simulink library "biogas"  (Simulink 7.8)
settings: Solver=ode45  StartTime=0.0  StopTime=10.0  RelTol=1e-3
undefined symbols (not defined in the file or in its folder): adm1_loadfcn, appendDATA, biogas, Callback_ADM1_gui, configdivider, configmixer, datasourcetypes, DEBUG, deltatime, gas2bhkwsplittypes, hydraulic_delay_loadfcn, init_biogas_plant_mdl, initstatetypes, kalman_loadfcn, lda_state_estimator_loadfcn, plant, plant_network, pump_energy_loadfcn, pump_stream_loadfcn, sensors, substrate, substrate_mixer_digester_loadfcn, substrate_network, volumeflowtypes
libraries: biogas x8, simulink x5
(part 1 of 2)
Description:
  | This library consists of blocks, which are useful for biogas plant modeling.
  | It belongs to the 'Biogas Plant Modeling' toolbox.
  | 
  | The library consists of seven sublibraries.
  | The most important blocks in these sublibraries are:
  | 
  | - Anaerobic Digestion Models
  | - Biogas Plant Components
  | - Commonly used blocks
  | - Optimization
  | - Sensors
  | - Simba Biogas Blocks
  | - Substrate Sources
settings Model: Creator=Daniel Gaida  LastModifiedBy=Daniel

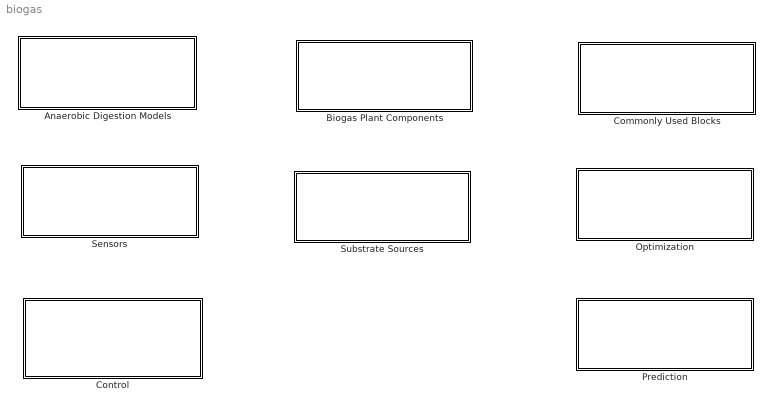
== system biogas ==
  Anaerobic Digestion Models : Subsystem  Description=This sub library contains blocks which model the anaerobic digestion process of a digester on a biogas plant. It includes the famous Anaerobic Digestion Model No.1 (ADM1).
      mask Type: Anaerobic Digestion Models
      mask Display: disp('Anaerobic Digestion Models')
  Biogas Plant Components : Subsystem  Description=This sub library contains blocks of components which are usually found on a biogas plant. Among these components are pump, heating, chp, mixer, etc...
      mask Type: Biogas Plant Components
      mask Display: disp('Biogas Plant Components')
  Commonly Used Blocks : Subsystem  Description=This sub library contains blocks, which are used very often modeling biogas plants.
      mask Type: Commonly Used Blocks
      mask Display: disp('Commonly Used Blocks')
  Control : Subsystem
      mask Display: disp('Control')
  Optimization : Subsystem
      mask Display: disp('Optimization')
  Prediction : Subsystem
      mask Display: disp('Prediction')
  Sensors : Subsystem  Description=This sub library contains measurement sensors, often installed on biogas plants.  mask(Sensors){d=0}
      mask help:
      | There is no public access to the Sensors using the Simulink Library Browser.
      | All sensors are integrated in other blocks, such as the ADM and substrate mixer blocks.
      mask Display: disp('Sensors')
  Substrate Sources : Subsystem
      mask Display: disp('Substrate Sources')

== system biogas/Anaerobic Digestion Models ==
  note: Callback_ADM1_gui('InitFcn', 'ADM1DE');
      | Callback_ADM1_gui('LoadFcn', 'ADM1DE');
      | Callback_ADM1_gui('ModelCloseFcn', 'ADM1DE');
      | Callback_ADM1_gui('StopFcn', 'ADM1DE');
  ADM1DE Linearized with GUI : Subsystem  LoadFcn=Callback_ADM1_gui('LoadFcn', 'ADM1DE', plant, DEBUG);  InitFcn=Callback_ADM1_gui('InitFcn', 'ADM1DE', plant, DEBUG);  StopFcn=Callback_ADM1_gui('StopFcn', 'ADM1DE', plant, DEBUG);  mask(ADM1 implementation with GUI (clone of Simba's ADM1xp model)){fermenter_name=--- Bitte Fermenter wählen ---, initstate_type=user, datasource_type=file, savestate=off, isload=off, isbeingloaded=off, isbeingclosed=off, DEBUG_DISP=off}
      mask prompts: fermenter_name "name of the fermenter (fermenter_name)"; initstate_type "initial state type (initstate_type)"; datasource_type "source for the initial state (datasource_type)"; savestate "save final state in variable/file (overwrite existing type, except default, than save in user)"; isload "if checked then this block is loaded"; isbeingloaded "if checked then this block is actually being loaded"; isbeingclosed "if checked then this block is actually being closed"; DEBUG_DISP "if checked then DEBUG_DISP modus is on for this block"
      mask help:
      | This block contains the block 'ADM1DE' and some measurement sensors like the pH, TS, SS, biogas and volumeflow sensor. These measurements are presented on a GUI, which is, in DEBUG mode, shown during the simulation.
      |
      | This block is implemented as the clone of the 'ADM1xp with GUI' block and can be used as an alternative, when Simba can't be used. For steady state simulations the gained results should be exactly the same.
      mask init:
      | if (DEBUG_DISP)
      |     disp(['Initialization commands of block ', gcb]);
      | end
      | 
      | values= get_param(gcb, 'MaskValues');
      | 
      | if isempty(values)
      |     error('Could not read the parameter MaskValues of block %s!', gcb);
      | end
      |     
      | if strcmp( char(values(5,1)), 'off' )
      | 
      |     if strcmp( char(values(6,1)), 'off' )
      |         
      |         if strcmp( char(values(7,1)), 'off' )
      |             
      |             Callback_ADM1_gui('LoadFcn', 'ADM1DE', plant, DEBUG, DEBUG_DISP);
      |             
      |         end
      |         
      |     end
      | 
      | else
      | 
      |     if strcmp( char(values(7,1)), 'off' )
      |             
      |         adm1_with_gui_setmasks(1,2,3,4);
      |         
      |     end
      | 
      | end
      | 
      | clear values;
      settings: ModelCloseFcn=Callback_ADM1_gui('ModelCloseFcn', 'ADM1DE', plant, DEBUG);
      mask StyleString: popup(--- Bitte Fermenter wählen ---),popup(--- Bitte Startzustandstyp wählen ---|default|random|user),popup(--- Bitte Datenquelle wählen ---|file|workspace|extern|modelworkspace),checkbox,checkbox,checkbox,checkbox,checkbox
      mask CallbackString:
      | values= get_param(gcb, 'MaskValues');
      | 
      | if isempty(values)
      |     error('Could not read the parameter MaskValues of block %s!', gcb);
      | end
      | 
      | if strcmp( char(values(5,1)), 'on' )
      | 
      |     display_selected_fermenter(1, 0.7);
      | 
      | end
      | 
      | clear values;
      | |
      | createinitstatetypepopup(2, 0);
      | |
      | createdatasourcetypepopup(3, 0);
      | |||||
      mask Display:
      | image(imread('icon_s6_digester','bmp'),'center')
      | port_label('input', 1, 'Qin', ...
      |     'texmode', 'on')
      | port_label('output', 1, 'Gas [m^3/d]')
      | port_label('output', 2, 'Qe')
      | port_label('output', 3, 'int.vars')
      | text(0.5, 7.0e-001, '--- Bitte Fermenter wählen ---', 'horizontalAlignment', 'center')
  ADM1DE with GUI : Subsystem  LoadFcn=Callback_ADM1_gui('LoadFcn', 'ADM1DE', plant, DEBUG);  InitFcn=Callback_ADM1_gui('InitFcn', 'ADM1DE', plant, DEBUG);  StopFcn=Callback_ADM1_gui('StopFcn', 'ADM1DE', plant, DEBUG);  mask(ADM1 implementation with GUI (clone of Simba's ADM1xp model)){fermenter_name=--- Bitte Fermenter wählen ---, initstate_type=user, datasource_type=file, savestate=off, isload=off, isbeingloaded=off, isbeingclosed=off, DEBUG_DISP=off, heating_onoff=off}
      mask prompts: fermenter_name "name of the fermenter (fermenter_name)"; initstate_type "initial state type (initstate_type)"; datasource_type "source for the initial state (datasource_type)"; savestate "save final state in variable/file (overwrite existing type, except default, than save in user)"; isload "if checked then this block is loaded"; isbeingloaded "if checked then this block is actually being loaded"; isbeingclosed "if checked then this block is actually being closed"; DEBUG_DISP "if checked then DEBUG_DISP modus is on for this block"; heating_onoff "check if heating is switched on, uncheck if digester is not heated"
      mask help:
      | This block contains the block 'ADM1DE' and some measurement sensors like the pH, TS, SS, biogas and volumeflow sensor. These measurements are presented on a GUI, which is, in DEBUG mode, shown during the simulation.
      |
      | This block is implemented as the clone of the 'ADM1xp with GUI' block and can be used as an alternative, when Simba can't be used. For steady state simulations the gained results should be exactly the same.
      mask init: same as biogas/Anaerobic Digestion Models/ADM1DE Linearized with GUI
      settings: ModelCloseFcn=Callback_ADM1_gui('ModelCloseFcn', 'ADM1DE', plant, DEBUG);
      mask StyleString: popup(--- Bitte Fermenter wählen ---),popup(--- Bitte Startzustandstyp wählen ---|default|random|user),popup(--- Bitte Datenquelle wählen ---|file|workspace|extern|modelworkspace),checkbox,checkbox,checkbox,checkbox,checkbox,checkbox
      mask CallbackString:
      | values= get_param(gcb, 'MaskValues');
      | 
      | if isempty(values)
      |     error('Could not read the parameter MaskValues of block %s!', gcb);
      | end
      | 
      | if strcmp( char(values(5,1)), 'on' )
      | 
      |     display_selected_fermenter(1, 0.7);
      | 
      | end
      | 
      | clear values;
      | |
      | createinitstatetypepopup(2, 0);
      | |
      | createdatasourcetypepopup(3, 0);
      | ||||||
      mask Display:
      | image(imread('icon_s6_digester','bmp'),'center')
      | port_label('input', 1, 'Qin', ...
      |     'texmode', 'on')
      | port_label('output', 1, 'Gas [m^3/d]')
      | port_label('output', 2, 'Qe')
      | text(0.5, 7.0e-001, '--- Bitte Fermenter wählen ---', 'horizontalAlignment', 'center')
  Internal : Subsystem
      mask Type: Internal Blocks
      mask Description: There is no public access to this group of blocks.
      mask Display: disp('No Public Access')

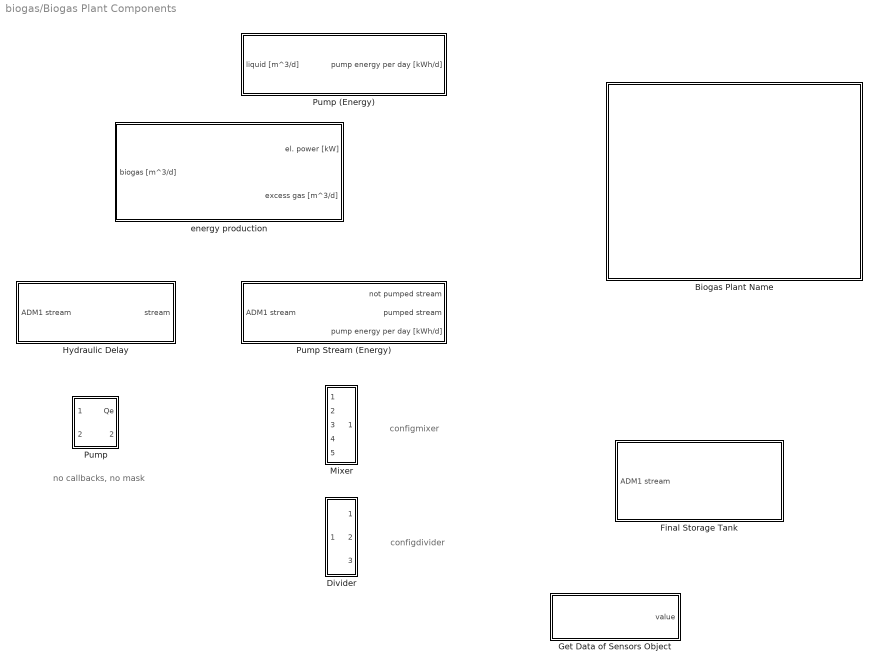
== system biogas/Biogas Plant Components ==
  note: no callbacks, no mask
  note: configmixer
  note: configdivider
  Biogas Plant Name : Subsystem  LoadFcn=init_biogas_plant_mdl();  InitFcn=init_biogas_plant_mdl();  mask(Biogas Plant    ){plant_name=plantname, debug=off, timegrid=min, timevalue=1}
      mask prompts: plant_name "Enter the name of the biogas plant (has to be identical with plant.name) (e.g. sunderhook):"; debug "Run model in DEBUG mode"; timegrid "In DEBUG mode much data is saved to file and workspace. Define here the unit of the timegrid"; timevalue "Select the number multiplied by the unit"
      mask help: This block serves as a framework for modeling your biogas plant. If you build a new biogas plant this block should be the first block you have to insert in the simulink model. Under the mask of this block you can then model your biogas plant by inserting digesters, chp's, substrate sources, pumps, etc...
      mask init:
      | values= get_param(gcb, 'MaskValues');
      | 
      | if ~isempty(values)
      | 
      |     img_filename= sprintf('plant_%s.jpg', char(values(1,1)));
      | 
      |     if ~exist(img_filename, 'file')
      |         warning(['Could not find the image ''', img_filename, ...
      |                 '''! Using the image ''plant_plantname.jpg'' instead!']);
      |         img_filename= 'plant_plantname.jpg';
      |     end
      |     
      | end
      mask StyleString: edit,checkbox,popup(day|hour|min|sec|each),popup(1)
      mask CallbackString:
      | init_biogas_plant_mdl();
      | |createtimevaluepopup();|createtimevaluepopup();|createtimevaluepopup();
      mask Display: image(imread(img_filename));
  Divider : Subsystem  InitFcn=configdivider();  mask(ADM1 Stream Divider){n_outputs=3, splitVector=[0.25, 0.5, 0.25, 0.1]}
      mask prompts: n_outputs "Number of Outflows"; splitVector "How should the stream be divided? Give a vector: e.g. [0.25, 0.5, 0.25], if number of Outputs = 3"
      mask help: This block divides the ADM1 stream.
      mask init:
      | %n_outputs=max(2,n_outputs);
      | if n_outputs == 1
      |     yi= 0.5;
      |     
      |     lb_x= 0;
      |     lb_y= -0.5;
      |     ub_x= 0.5;
      |     ub_y= 1.5;
      | else
      |     yi=[0:n_outputs-1]/(n_outputs-1);
      |     
      |     lb_x= 0;
      |     lb_y= -0.5/(n_outputs-1);
      |     ub_x= 0.5;
      |     ub_y= 1 + 0.5/(n_outputs-1);
      | end
      | 
      | x=[];y=[];
      | 
      | for i=1:n_outputs,
      |    
      |     x=[x; 0.0;0.3; 0.5;0.3; 0.0];
      |     y=[y;0.5; yi(i);yi(i);yi(i);0.5];
      |   
      | end;
      | 
      | configdivider();
      mask Help: eval('web( ''html/divider.html'', ''-helpbrowser'')')
      mask Display: plot(lb_x, lb_y, ub_x, ub_y, x, y);
  Final Storage Tank : Subsystem
      mask Type: Final Storage Tank
      mask Description: This block models the final storage tank.
      mask Display:
      | image(imread('images/final_storage_tank.bmp'))
      | color('red')
      | 
      | port_label('input', 1, 'ADM1 stream')
  Get Data of Sensors Object : Subsystem  mask(Get Data of Sensors Object){processvalue='Q_main_2', id_in_array='', index=0, noisy=off}
      mask prompts: processvalue "process value id"; index "index in sensor (0, 1, 2, ...)"; noisy "noisy sensor values"
      mask help: This block returns the current value of the specified process value.
      settings: AttributesFormatString=%<processvalue>
  Hydraulic Delay : Subsystem  LoadFcn=hydraulic_delay_loadfcn();  mask(Hydraulic Delay){fermenter_name_start=--- Bitte Fermenter wählen ---, fermenter_name_destiny=--- Bitte Fermenter wählen ---, initstate_type=--- Bitte Startzustandstyp wählen ---, datasource_type=--- Bitte Datenquelle wählen ---, savestate=off, time_constant=10, V_min=100, isload=on, isbeingloaded=off, isbeingclosed=off, DEBUG_DISP=off}
      mask prompts: fermenter_name_start "name of the start fermenter (fermenter_name_start)"; fermenter_name_destiny "name of the destiny fermenter (fermenter_name_destiny)"; initstate_type "initial state type (initstate_type)"; datasource_type "source for the initial state (datasource_type)"; savestate "save final state in variable/file (overwrite existing type, except default, than save in user)"; time_constant "Time constant [d]"; V_min "Minimum Volume [m^3]"; isload "if checked then this block is loaded"; isbeingloaded "if checked then this block is actually being loaded"; isbeingclosed "if checked then this block is actually being closed"; DEBUG_DISP "if checked then DEBUG_DISP modus is on for this block"
      mask help:
      | This block implements a hydraulic delay (first order storage).
      |
      | It is mainly used to avoid numerical loops. Most of the time they appear when substrate is pumped in a loop. Out of this reason the block 'Pump Stream (Energy)' consists this hydraulic delay block, such that, if you want to pump substrate in a loop, you don't have to bother about numerical loops. To summarize, normally you don't have to use this block.
      mask init:
      | x=[0:5:50];
      | y=ones(1,size(x,1))-exp(-x/5);
      | y=y*70;
      | 
      | 
      | if ~isempty(bdroot)
      |     hws= get_param(bdroot, 'modelworkspace');
      | else
      |     hws= [];
      | end
      | 
      | if ~isempty(hws)
      |    
      | if DEBUG_DISP       
      |     disp(['Initialization commands of block ', gcb]);
      | end
      | 
      | values= get_param(gcb, 'MaskValues');
      | 
      | if isempty(values)
      |     error('Could not read the parameter MaskValues of block %s!', gcb);
      | end
      |     
      | if strcmp( char(values(8,1)), 'off' )
      | 
      |     if strcmp( char(values(9,1)), 'off' )
      |         
      |         if strcmp( char(values(10,1)), 'off' )
      |          
      |             hydraulic_delay_loadfcn(DEBUG_DISP);
      |             
      |         end
      |         
      |     end
      | 
      | end
      | 
      | end
      | 
      | clear values hws;
      settings: ModelCloseFcn=hydraulic_delay_closefcn();
      mask Help: eval('web( ''html/hydraulic_delay.html'', ''-helpbrowser'')')
      mask StyleString: popup(--- Bitte Fermenter wählen ---),popup(--- Bitte Fermenter wählen ---),popup(--- Bitte Startzustandstyp wählen ---|default|random|user),popup(--- Bitte Datenquelle wählen ---|file|workspace|extern|modelworkspace),checkbox,edit,edit,checkbox,checkbox,checkbox,checkbox
      mask CallbackString:
      | values= get_param(gcb, 'MaskValues');
      | 
      | if isempty(values)
      |     error('Could not read the parameter MaskValues of block %s!', gcb);
      | end
      | 
      | if strcmp( char(values(8,1)), 'on' )
      | 
      |     display_selected_fermenter(1, 0.8);
      | 
      | end
      | 
      | clear values;
      | |
      | values= get_param(gcb, 'MaskValues');
      | 
      | if isempty(values)
      |     error('Could not read the parameter MaskValues of block %s!', gcb);
      | end
      | 
      | if strcmp( char(values(8,1)), 'on' )
      | 
      |     display_selected_fermenter(2, 0.4);
      | 
      | end
      | 
      | clear values;
      | |
      | values= get_param(gcb, 'MaskValues');
      | 
      | if isempty(values)
      |     error('Could not read the parameter MaskValues of block %s!', gcb);
      | end
      | 
      | if strcmp( char(values(8,1)), 'on' )
      | 
      |     createvolumeflowtypepopup(3, 0);
      | 
      | end
      | 
      | clear values;
      | |
      | values= get_param(gcb, 'MaskValues');
      | 
      | if isempty(values)
      |     error('Could not read the parameter MaskValues of block %s!', gcb);
      | end
      | 
      | if strcmp( char(values(8,1)), 'on' )
      | 
      |     createdatasourcetypepopup(4, 0);
      | 
      | end
      | 
      | clear values;
      | |||||||
      mask Display:
      | plot(0,0,100,100,[15,15,85],[85,15,15],...
      |      x+15,y+15,[0,10],[15,0]);
      |  text(0.5, 8.0e-001, '--- Bitte Fermenter wählen ---', 'horizontalAlignment', 'center')
      |  text(0.5, 4.0e-001, '--- Bitte Fermenter wählen ---', 'horizontalAlignment', 'center')
  Mixer : Subsystem  InitFcn=configmixer();  mask(Substrate Mixer){n_inputs=5}
      mask prompts: n_inputs "Number of Inflows"
      mask help: This block mixes the substrate flow.
      mask init:
      | %n_inputs=max(2,n_inputs);
      | 
      | if n_inputs == 1
      |     yi= 0.5;
      |     
      |     lb_x= 0;
      |     lb_y= -0.5;
      |     ub_x= 0.5;
      |     ub_y= 1.5;
      | else
      |     yi=[0:n_inputs-1]/(n_inputs-1);
      |     
      |     lb_x= 0;
      |     lb_y= -0.5/(n_inputs-1);
      |     ub_x= 0.5;
      |     ub_y= 1+0.5/(n_inputs-1);
      | end
      | 
      | x=[];y=[];
      | for i=1:n_inputs,
      |    
      |     x=[x; 0.5;0.2; 0.0;0.2; 0.5];
      |     y=[y;0.5; yi(i);yi(i);yi(i);0.5];
      |   
      | end;
      | 
      | configmixer();
      mask Help: eval('web( ''html/mixer.html'', ''-helpbrowser'')')
      mask Display: plot(lb_x, lb_y, ub_x, ub_y, x, y);
  Pump : Subsystem  mask(Pump){}
      mask help:
      | Pump a separated substrate stream flow.
      |
      | Remark: For the most purposes the 'Pump Stream (Energy)' block should be a better alternative.
      mask init:
      | x1=[10,90];
      | y1=[75,75];
      | x2=[30,40];
      | y2=[75,65];
      | x3=[65,80,90];
      | y3=[40,25,25];
      | 
      | ori=get_param(gcb,'orientation');
      | 
      | if strcmp(ori,'left')
      |     x1=100-x1;
      |     x2=100-x2;
      |     x3=100-x3;
      | elseif strcmp(ori,'down')
      |     xt=x1;
      |     x1=100-y1;
      |     y1=100-xt;
      |     xt=x2;
      |     x2=100-y2;
      |     y2=100-xt;
      |     xt=x3;
      |     x3=100-y3;
      |     y3=100-xt;
      | elseif strcmp(ori,'up')
      |     xt=x1;
      |     x1=100-y1;
      |     y1=xt;
      |     xt=x2;
      |     x2=100-y2;
      |     y2=xt;
      |     xt=x3;
      |     x3=100-y3;
      |     y3=xt;
      | end
      mask Display: plot(0,0,100,100,x1,y1,x2,y2,x3,y3,[0,20],[20,0]);disp('P')
  Pump (Energy) : Subsystem  LoadFcn=pump_energy_loadfcn();  mask(Pump (Energy)){fermenter_name=--- Bitte Fermenter wählen ---, h_friction=1.0, isload=off, isbeingloaded=off, isbeingclosed=off, DEBUG_DISP=off}
      mask prompts: fermenter_name "name of the fermenter (fermenter_name)"; isload "if checked then this block is loaded"; isbeingloaded "if checked then this block is actually being loaded"; isbeingclosed "if checked then this block is actually being closed"; DEBUG_DISP "if checked then DEBUG_DISP modus is on for this block"
      mask help:
      | This block calculates the power used to pump the substrate mix, whose volumeflow is given on the input.
      |
      | Remark: If you want to pump a stream, then use the block 'Pump' or even better the block 'Pump Stream (Energy)'.
      mask init:
      | if DEBUG_DISP
      |     disp(['Initialization commands of block ', gcb]);
      | end
      | 
      | values= get_param(gcb, 'MaskValues');
      | 
      | if isempty(values)
      |     error('Could not read the parameter MaskValues of block %s!', gcb);
      | end
      |     
      | if strcmp( char(values(3,1)), 'off' )
      | 
      |     if strcmp( char(values(4,1)), 'off' )
      |         
      |         if strcmp( char(values(5,1)), 'off' )
      |          
      |             pump_energy_loadfcn(DEBUG_DISP);
      |             
      |         end
      |         
      |     end
      | 
      | end
      | 
      | clear values;
      settings: ModelCloseFcn=pump_energy_closefcn();
      mask Help: eval('web( ''html/pump.html'', ''-helpbrowser'')')
      mask StyleString: popup(--- Bitte Fermenter wählen ---),edit,checkbox,checkbox,checkbox,checkbox
      mask CallbackString:
      | values= get_param(gcb, 'MaskValues');
      | 
      | if isempty(values)
      |     error('Could not read the parameter MaskValues of block %s!', gcb);
      | end
      | 
      | if strcmp( char(values(3,1)), 'on' )
      | 
      |     display_selected_fermenter(1, 0.3);
      | 
      | end
      | 
      | clear values;
      | 
      | |||||
      mask Display:
      | image(imread('images/Pumpe.jpg'))
      | color('red')
      | 
      | port_label('input', 1, 'liquid [m^3/d]', ...
      |     'texmode', 'on')
      | port_label('output', 1, 'pump energy per day [kWh/d]')
  Pump Stream (Energy) : Subsystem  LoadFcn=pump_stream_loadfcn();  mask(Pump Stream (Energy)){fermenter_name_start=--- Bitte Fermenter wählen ---, fermenter_name_destiny=--- Bitte Fermenter wählen ---, volumeflow_type=const, datasource_type=workspace, h_friction=1.0, hyd_delay=on, initstate_type=default, savestate=on, time_constant=1/24/30, V_min=100, isload=off, isbeingloaded=off, isbeingclosed=off, DEBUG_DISP=off}
      mask prompts: fermenter_name_start "name of the start fermenter (fermenter_name_start)"; fermenter_name_destiny "name of the destiny fermenter (fermenter_name_destiny)"; volumeflow_type "volumeflow_type : type of the volume flow pump data"; datasource_type "source for the volumeflow (datasource_type)"; hyd_delay "avoid algebraic loop by inserting an hydraulic delay"; initstate_type "initial state type (initstate_type)"; savestate "save final state in variable/file (overwrite existing type, except default, then save in user)"; time_constant "Time constant [d]"; V_min "Minimum Volume [m^3]"; isload "if checked then this block is loaded"; isbeingloaded "if checked then this block is actually being loaded"; isbeingclosed "if checked then this block is actually being closed"; DEBUG_DISP "if checked then DEBUG_DISP modus is on for this block"
      mask help: This block pumps a substrate stream and calculates the power used to pump the substrate stream. To avoid numerical loops this block contains the 'Hydraulic Delay' block, which can be inserted or deleted via the gui of this block.
      mask init:
      | pump_stream_init_comm(DEBUG_DISP);
      settings: ModelCloseFcn=pump_stream_closefcn();
      mask Help: eval('web( ''html/pump_stream.html'', ''-helpbrowser'')')
      mask StyleString: popup(--- Bitte Fermenter wählen ---),popup(--- Bitte Fermenter wählen ---),popup(--- Bitte Zulauftyp wählen ---|const|random|user),popup(--- Bitte Datenquelle wählen ---|file|workspace|extern|modelworkspace),edit,checkbox,popup(--- Bitte Startzustandstyp wählen ---|default|random|user),checkbox,edit,edit,checkbox,checkbox,checkbox,checkbox
      mask CallbackString:
      | values= get_param(gcb, 'MaskValues');
      | 
      | if isempty(values)
      |     error('Could not read the parameter MaskValues of block %s!', gcb);
      | end
      | 
      | if strcmp( char(values(11,1)), 'on' )
      | 
      |     display_selected_fermenter(1, 0.8);
      | 
      | end
      | 
      | clear values;
      | |
      | values= get_param(gcb, 'MaskValues');
      | 
      | if isempty(values)
      |     error('Could not read the parameter MaskValues of block %s!', gcb);
      | end
      | 
      | if strcmp( char(values(11,1)), 'on' )
      | 
      |     display_selected_fermenter(2, 0.4);
      | 
      | end
      | 
      | clear values;
      | |
      | values= get_param(gcb, 'MaskValues');
      | 
      | if isempty(values)
      |     error('Could not read the parameter MaskValues of block %s!', gcb);
      | end
      | 
      | if strcmp( char(values(11,1)), 'on' )
      | 
      |     createvolumeflowtypepopup(3, 0);
      | 
      | end
      | 
      | clear values;
      | |
      | values= get_param(gcb, 'MaskValues');
      | 
      | if isempty(values)
      |     error('Could not read the parameter MaskValues of block %s!', gcb);
      | end
      | 
      | if strcmp( char(values(11,1)), 'on' )
      | 
      |     createdatasourcetypepopup(4, 0);
      | 
      | end
      | 
      | clear values;
      | ||pump_stream_eval_loop_check(6);|
      | values= get_param(gcb, 'MaskValues');
      | 
      | if isempty(values)
      |     error('Could not read the parameter MaskValues of block %s!', gcb);
      | end
      | 
      | if strcmp( char(values(11,1)), 'on' )
      | 
      |     createinitstatetypepopup(7, 0);
      | 
      | end
      | 
      | clear values;
      |   |||||||
      mask Display:
      | image(imread('images/Pumpe.jpg'))
      | color('red')
      | 
      | port_label('input', 1, 'ADM1 stream')
      | port_label('output', 1, 'not pumped stream')
      | port_label('output', 2, 'pumped stream')
      | port_label('output', 3, 'pump energy per day [kWh/d]')
  energy production : Subsystem  LoadFcn=|  mask(Biogas Distributor){gas2bhkwsplit_type=--- Bitte Splittyp wählen ---}
      | set_param(gcb, 'UserDataPersistent', 'on')
      |                                           
      | creategas2bhkwsplittypepopup(1, 1);
      mask prompts: gas2bhkwsplit_type "type of splitting gas (gas2bhkwsplittype)"
      mask help: This block distributes the biogas flow to the biogas chp's on the plant. How the biogas should be distributed can be chosen via the block's gui.
      settings: AttributesFormatString=splittype= %<gas2bhkwsplit_type>
      mask Help: eval('web(''html/biogas2bhkw.html'', ''-helpbrowser'')')
      mask StyleString: popup(--- Bitte Splittyp wählen ---|fiftyfifty|one2one|threshold)
      mask CallbackString: creategas2bhkwsplittypepopup(1, 0);
      mask Display:
      | image(imread('images/jenbacher.jpg'))
      | color('red')
      | port_label('input', 1, 'biogas [m^3/d]', ...
      |     'texmode', 'on')
      | port_label('output', 1, 'el. power [kW]', ...
      |     'texmode', 'on')
      | port_label('output', 2, 'excess gas [m^3/d]', ...
      |     'texmode', 'on')

== system biogas/Commonly Used Blocks ==
  ADM1DE with GUI : biogas/Anaerobic Digestion Models/ADM1DE with GUI  fermenter_name=--- Bitte Fermenter wählen ---  initstate_type=user  datasource_type=file  savestate=off  isload=off  isbeingloaded=off  isbeingclosed=off  DEBUG_DISP=off  heating_onoff=off
  Biogas Plant Name : biogas/Biogas Plant Components/Biogas Plant Name  plant_name=plantname  debug=off  timegrid=min  timevalue=1
  Mixer : biogas/Biogas Plant Components/Mixer  n_inputs=5
  Pump Stream (Energy) : biogas/Biogas Plant Components/Pump Stream (Energy)  fermenter_name_start=--- Bitte Fermenter wählen ---  fermenter_name_destiny=--- Bitte Fermenter wählen ---  volumeflow_type=const  datasource_type=workspace  h_friction=1.0  hyd_delay=on  initstate_type=default  savestate=on  time_constant=1/24/30  V_min=100  isload=off  isbeingloaded=off  isbeingclosed=off  DEBUG_DISP=off
  Substrate Mixer (Digester) : biogas/Substrate Sources/Substrate Mixer (Digester)  volumeflow_type=const  datasource_type=file  error=0.0  isload=off  isbeingloaded=off  isbeingclosed=off  DEBUG_DISP=off
      settings: AttributesFormatString=q= %<volumeflow_type>

== system biogas/Control ==
  CH4 SP Control Antonelli : Subsystem  mask(CH4 setpoint control by Antonelli 2002){kch4=0.075, manual=off}
      mask prompts: manual "manual operation (Handbetrieb) (ref is passed through)"
      mask help:
      | Methane setpoint control:
      |
      | D= kch4 * (D - Dmax) * (D - Dmin) * (Qch4 - Qch4ref)
      |
      | Dmin and Dmax as given
  CH4 SP Control Antonelli Dmin < Dref < Dmax : Subsystem  mask(CH4 setpoint control by Antonelli 2002){kch4=0.075, Dslope=0.25, manual=off}
      mask prompts: Dslope "Dslope [100 %]"; manual "manual operation (Handbetrieb) (ref is passed through)"
      mask help:
      | Methane setpoint control:
      |
      | D= kch4 * (D - Dmax) * (D - Dmin) * (Qch4 - Qch4ref)
      |
      | Dmin= (1 - Dslope) * Dref
      | Dmax= (1 + Dslope) * Dref
  CH4 SP Control Antonelli Dmin < Dref < Dmax change of D as absolute value : Subsystem  mask(CH4 setpoint control by Antonelli 2002){kch4=0.075, Dchange=0.05, manual=off}
      mask prompts: Dchange "Dchange [1/d]"; manual "manual operation (Handbetrieb) (ref is passed through)"
      mask help:
      | Methane setpoint control:
      |
      | D= kch4 * (D - Dmax) * (D - Dmin) * (Qch4 - Qch4ref)
      |
      | Dmin= Dref - Dchange
      | Dmax= Dref + Dchange
  CH4 SP Control Antonelli Dmin < Dref < Dmax extended by Gaida : Subsystem  mask(CH4 setpoint control by Antonelli 2002){kch4=0.075, kch4rel=0, Dchange=0.05, manual=off}
      mask prompts: Dchange "Dchange [1/d]"; manual "manual operation (Handbetrieb) (ref is passed through)"
      mask help:
      | Methane setpoint control:
      |
      | D= kch4 * (D - Dmax) * (D - Dmin) * (Qch4 - Qch4ref)
      |
      | Dmin= Dref - Dchange
      | Dmax= Dref + Dchange
  CH4 SP Control Antonelli Dmin < Dref < Dmax extended by Gaida 2nd : Subsystem  mask(CH4 setpoint control by Antonelli 2002){kch4=0.075, kch4rel=0, Dchange=0.05, manual=off}
      mask prompts: Dchange "Dchange [1/d]"; manual "manual operation (Handbetrieb) (ref is passed through)"
      mask help:
      | Methane setpoint control:
      |
      | D= kch4 * (D - Dmax) * (D - Dmin) * (Qch4 - Qch4ref)
      |
      | Dmin= Dref - Dchange
      | Dmax= Dref + Dchange

== system biogas/Optimization ==
  fitness sensor : Subsystem
      mask Type: database sink
      mask Description: This block saves the individual in a database.
      mask Help: eval('web( ''html/database_write.html'', ''-helpbrowser'')')
      mask Display: port_label('output', 1, 'fitness')
  simulation killer : Subsystem
      mask Type: simulation killer
      mask Description: This block terminates the simulation after a given time has past.
      mask Help: eval('web( ''html/kill_simulation.html'', ''-helpbrowser'')')

== system biogas/Prediction ==
  Kalman Filter cont. : Subsystem  LoadFcn=kalman_loadfcn();  mask(Continuous Kalman filter as DE system){fermenter_name=--- Bitte Fermenter wählen ---, initstate_type=--- Bitte Startzustandstyp wählen ---, datasource_type=--- Bitte Datenquelle wählen ---, isload=off, isbeingloaded=off, isbeingclosed=off, DEBUG_DISP=off}
      mask prompts: fermenter_name "name of the fermenter (fermenter_name)"; initstate_type "initial state type (initstate_type)"; datasource_type "source for the initial state (datasource_type)"; isload "if checked then this block is loaded"; isbeingloaded "if checked then this block is actually being loaded"; isbeingclosed "if checked then this block is actually being closed"; DEBUG_DISP "if checked then DEBUG_DISP modus is on for this block"
      mask init:
      | if DEBUG_DISP
      |     disp(['Initialization commands of block ', gcb]);
      | end
      | 
      | values= get_param(gcb, 'MaskValues');
      | 
      | if isempty(values)
      |     error('Could not read the parameter MaskValues of block %s!', gcb);
      | end
      |     
      | if strcmp( char(values(4,1)), 'off' )
      | 
      |     if strcmp( char(values(5,1)), 'off' )
      |         
      |         if strcmp( char(values(6,1)), 'off' )
      |          
      |             kalman_loadfcn(DEBUG_DISP);
      |             
      |         end
      |         
      |     end
      | 
      | end
      | 
      | clear values;
      settings: ModelCloseFcn=kalman_closefcn();
      mask Help: eval('web( ''html/KalmanFilterContinuous.html'', ''-helpbrowser'')')
      mask StyleString: popup(--- Bitte Fermenter wählen ---),popup(--- Bitte Startzustandstyp wählen ---|default|random|user),popup(--- Bitte Datenquelle wählen ---|file|workspace|extern|modelworkspace),checkbox,checkbox,checkbox,checkbox
      mask CallbackString:
      | values= get_param(gcb, 'MaskValues');
      | 
      | if isempty(values)
      |     error('Could not read the parameter MaskValues of block %s!', gcb);
      | end
      | 
      | if strcmp( char(values(5,1)), 'on' )
      | 
      |     display_selected_fermenter(1, 0.7);
      | 
      | end
      | 
      | clear values;
      | |createinitstatetypepopup(2, 0);
      | |createdatasourcetypepopup(3, 0);
      | ||||
      mask Display:
      | port_label('input',1,'Qin')
      | port_label('output',1,'x hat')
      | text(0.5, 7.0e-001, '--- Bitte Fermenter wählen ---', 'horizontalAlignment', 'center')
  LDA State Estimator : Subsystem  LoadFcn=lda_state_estimator_loadfcn();  mask(LDA State Estimator){fermenter_name=--- Bitte Fermenter wählen ---, isload=off, isbeingloaded=off, isbeingclosed=off, DEBUG_DISP=off}
      mask prompts: fermenter_name "name of the fermenter (fermenter_name)"; isload "if checked then this block is loaded"; isbeingloaded "if checked then this block is actually being loaded"; isbeingclosed "if checked then this block is actually being closed"; DEBUG_DISP "if checked then DEBUG_DISP modus is on for this block"
      mask help: This block estimates the state of the selected fermenter.
      mask init:
      | if DEBUG_DISP
      |     disp(['Initialization commands of block ', gcb]);
      | end
      | 
      | values= get_param(gcb, 'MaskValues');
      | 
      | if isempty(values)
      |     error('Could not read the parameter MaskValues of block %s!', gcb);
      | end
      |     
      | if strcmp( char(values(2,1)), 'off' )
      | 
      |     if strcmp( char(values(3,1)), 'off' )
      |         
      |         if strcmp( char(values(4,1)), 'off' )
      |          
      |             lda_state_estimator_loadfcn(DEBUG_DISP);
      |             
      |         end
      |         
      |     end
      | 
      | end
      | 
      | clear values;
      settings: ModelCloseFcn=lda_state_estimator_closefcn();
      mask Help: eval('web( ''html/LDAStateEstimator.html'', ''-helpbrowser'')')
      mask StyleString: popup(--- Bitte Fermenter wählen ---),checkbox,checkbox,checkbox,checkbox
      mask CallbackString:
      | values= get_param(gcb, 'MaskValues');
      | 
      | if isempty(values)
      |     error('Could not read the parameter MaskValues of block %s!', gcb);
      | end
      | 
      | if strcmp( char(values(2,1)), 'on' )
      | 
      |     display_selected_fermenter(1, 0.7);
      | 
      | end
      | 
      | clear values;
      | 
      | ||||
      mask Display: port_label('output', 1, 'state estimate')
  RF State Estimator : Subsystem  LoadFcn=lda_state_estimator_loadfcn();  mask(RF State Estimator){fermenter_name=--- Bitte Fermenter wählen ---, isload=off, isbeingloaded=off, isbeingclosed=off, DEBUG_DISP=off}
      mask prompts: fermenter_name "name of the fermenter (fermenter_name)"; isload "if checked then this block is loaded"; isbeingloaded "if checked then this block is actually being loaded"; isbeingclosed "if checked then this block is actually being closed"; DEBUG_DISP "if checked then DEBUG_DISP modus is on for this block"
      mask help: This block estimates the state of the selected fermenter using Random Forests.
      mask init: same as biogas/Prediction/LDA State Estimator
      settings: ModelCloseFcn=lda_state_estimator_closefcn();
      mask Help: eval('web( ''html/RFStateEstimator.html'', ''-helpbrowser'')')
      mask StyleString: popup(--- Bitte Fermenter wählen ---),checkbox,checkbox,checkbox,checkbox
      mask CallbackString:
      | values= get_param(gcb, 'MaskValues');
      | 
      | if isempty(values)
      |     error('Could not read the parameter MaskValues of block %s!', gcb);
      | end
      | 
      | if strcmp( char(values(2,1)), 'on' )
      | 
      |     display_selected_fermenter(1, 0.7);
      | 
      | end
      | 
      | clear values;
      | 
      | ||||
      mask Display: port_label('output', 1, 'state estimate')

== system biogas/Sensors ==
  note: no callbacks, no mask
  note: TODO:
      | SRT Sensor implementieren
      | gesamte substratzufuhr
      | zu gesamtvolumen
  substrateflow sensor : Subsystem  mask(Substrate flow sensor){}
      mask help: Substrate flow measurement sensor [m^3/d].
      mask init:
      | x=50+50*sin(0:0.1:2*pi+0.2);
      | y=50+50*cos(0:0.1:2*pi+0.2);
      mask Help: Selects the 34th component out of the ADM1xp vector stream.
      mask Display:
      | plot(0,0,100,100,x,y);
      | disp('F')

== system biogas/Substrate Sources ==
  Internal : Subsystem  mask(No Public Access){internal=off}
      mask help:
      | You can not access the content of this group using the Simulink Library.
      | In this group only those blocks are located, which are used internally in the toolbox. So there is no need to get access to them.
      mask Display: disp('No Public Access')
  Substrate Mixer (Digester) : Subsystem  LoadFcn=substrate_mixer_digester_loadfcn();  mask(Substrate Mixer (Digester)){volumeflow_type=const, datasource_type=file, error=0.0, isload=off, isbeingloaded=off, isbeingclosed=off, DEBUG_DISP=off}
      mask prompts: volumeflow_type "volumeflow_type : type of the volume flow input data"; datasource_type "source for the volumeflow (datasource_type)"; error "error : value of noise, desturbing the primary data [100 %]"; isload "if checked then this block is loaded"; isbeingloaded "if checked then this block is actually being loaded"; isbeingclosed "if checked then this block is actually being closed"; DEBUG_DISP "if checked then DEBUG_DISP modus is on for this block"
      mask help: This block creates the substrate mix for each fermenter. The mix is constructed by mixing the streams of the 'Substrate Source (Digester)' blocks.
      mask init:
      | %%
      | % 
      | 
      | if ~isempty(bdroot)
      |     hws= get_param(bdroot, 'modelworkspace');
      | else
      |     hws= [];
      | end
      | 
      | if isempty(hws)
      |    return; 
      | end
      | 
      | if DEBUG_DISP
      |     disp(['Initialization commands of block ', gcb]);
      | end
      | 
      | values= get_param(gcb, 'MaskValues');
      | 
      | if isempty(values)
      |     error('Could not read the parameter MaskValues of block %s!', gcb);
      | end
      | 
      | if strcmp( char(values(4,1)), 'off' )
      | 
      |     if strcmp( char(values(5,1)), 'off' )
      |         
      |         if strcmp( char(values(6,1)), 'off' )
      |             
      |             substrate_mixer_digester_loadfcn(DEBUG_DISP);
      |             
      |         end
      |         
      |     end
      | 
      | else
      |     
      |     if strcmp( char(values(6,1)), 'off' )
      |             
      |         substrate_mixer_digester_init_commands(DEBUG_DISP);
      |         
      |     end
      | 
      | end
      | 
      | clear values hws;
      settings: AttributesFormatString=q= %<volumeflow_type>  ModelCloseFcn=substrate_mixer_digester_closefcn();
      mask StyleString: popup(--- Bitte Zulauftyp wählen ---|const|random|user),popup(--- Bitte Datenquelle wählen ---|file|workspace|extern|modelworkspace),edit,checkbox,checkbox,checkbox,checkbox
      mask CallbackString:
      | createvolumeflowtypepopup(1, 0);
      |     |createdatasourcetypepopup(2, 0);
      |     |||||
      mask Display: image(imread('images/Substrate_feed.jpg'))

== system biogas/Anaerobic Digestion Models/ADM1DE Linearized with GUI ==
  Qin : Inport
  combi - ADM1xp digester : biogas/Anaerobic Digestion Models/Internal/ADM1DE Linearized  fermenter_name=--- Bitte Fermenter wählen ---  initstate_type=user  datasource_type=file  savestate=off  isload=off  isbeingloaded=off  isbeingclosed=off  DEBUG_DISP=off
  Gas [m³/d] : Outport
  Qe : Outport  Port=2
  int.vars : Outport  Port=3
  wires:
  combi - ADM1xp digester/1 -> Gas [m³/d]/1
  Qin/1 -> combi - ADM1xp digester/1
  combi - ADM1xp digester/2 -> Qe/1
  combi - ADM1xp digester/3 -> int.vars/1

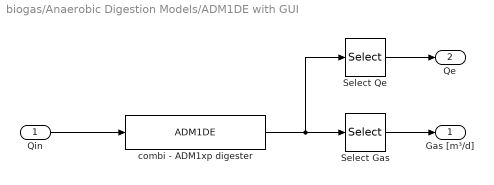
== system biogas/Anaerobic Digestion Models/ADM1DE with GUI ==
  Qin : Inport
  Select Gas : Selector  InputPortWidth=biogas.ADMstate.dim_stream + biogas.BioGas.n_gases  IndexOptions=Index vector (dialog)  Indices=[35:37]  OutputSizes=1
  Select Qe : Selector  InputPortWidth=biogas.ADMstate.dim_stream + biogas.BioGas.n_gases  IndexOptions=Index vector (dialog)  Indices=[1:biogas.ADMstate.dim_stream]  OutputSizes=1
  combi - ADM1xp digester : S-Function  FunctionName=ADM1DE  Parameters=sensors, plant, substrate, substrate_network, plant_network, char(plant.getDigesterID(fermenter_name - 1)), initstatetypes(initstate_type - 1), datasourcetypes(datasource_type - 1), savestate, heating_onoff  EnableBusSupport=off
  Gas [m³/d] : Outport
  Qe : Outport  Port=2
  wires:
  Select Qe/1 -> Qe/1
  Qin/1 -> combi - ADM1xp digester/1
  Select Gas/1 -> Gas [m³/d]/1
  combi - ADM1xp digester/1 -> Select Qe/1, Select Gas/1

== system biogas/Anaerobic Digestion Models/Internal ==
  note: adm1_loadfcn('ADM1DE');
      | adm1_closefcn('ADM1DE');
  note: these blocks are not used anymore as it seems to me
  ADM1DE : Subsystem  LoadFcn=adm1_loadfcn('ADM1DE');  mask(ADM1 implemented as DE system){fermenter_name=--- Bitte Fermenter wählen ---, initstate_type=--- Bitte Startzustandstyp wählen ---, datasource_type=--- Bitte Datenquelle wählen ---, savestate=off, isload=off, isbeingloaded=off, isbeingclosed=off, DEBUG_DISP=off}
      mask prompts: fermenter_name "name of the fermenter (fermenter_name)"; initstate_type "initial state type (initstate_type)"; datasource_type "source for the initial state (datasource_type)"; savestate "save final state in variable/file (overwrite existing type, except default, than save in user)"; isload "if checked then this block is loaded"; isbeingloaded "if checked then this block is actually being loaded"; isbeingclosed "if checked then this block is actually being closed"; DEBUG_DISP "if checked then DEBUG_DISP modus is on for this block"
      mask help:
      | This block is an implementation of the ADM1 as DE system as a clone of Simba's ADM1xp model.
      |
      | Remark: It is recommended to use the 'ADM1DE with GUI' block instead of this one, because the other block contains already measurement sensors, whose measurments are shown on a GUI.
      mask init:
      | if DEBUG_DISP
      |     disp(['Initialization commands of block ', gcb]);
      | end
      | 
      | values= get_param(gcb, 'MaskValues');
      | 
      | if isempty(values)
      |     error('Could not read the parameter MaskValues of block %s!', gcb);
      | end
      |     
      | if strcmp( char(values(5,1)), 'off' )
      | 
      |     if strcmp( char(values(6,1)), 'off' )
      |         
      |         if strcmp( char(values(7,1)), 'off' )
      |          
      |             adm1_loadfcn('ADM1DE', DEBUG_DISP);
      |             
      |         end
      |         
      |     end
      | 
      | end
      | 
      | clear values;
      settings: ModelCloseFcn=adm1_closefcn('ADM1DE');
      mask Help: eval('web( ''html/ADM1DE.html'', ''-helpbrowser'')')
      mask StyleString: popup(--- Bitte Fermenter wählen ---),popup(--- Bitte Startzustandstyp wählen ---|default|random|user),popup(--- Bitte Datenquelle wählen ---|file|workspace|extern|modelworkspace),checkbox,checkbox,checkbox,checkbox,checkbox
      mask CallbackString:
      | values= get_param(gcb, 'MaskValues');
      | 
      | if isempty(values)
      |     error('Could not read the parameter MaskValues of block %s!', gcb);
      | end
      | 
      | if strcmp( char(values(5,1)), 'on' )
      | 
      |     display_selected_fermenter(1, 0.7);
      | 
      | end
      | 
      | clear values;
      | |createinitstatetypepopup(2, 0);
      | |createdatasourcetypepopup(3, 0);
      | |||||
      mask Display:
      | image(imread('icon_s6_digester','bmp'),'center')
      | 
      | port_label('input',1,'Qin')
      | port_label('output',1,'Gas')
      | port_label('output',2,'Qe')
      | text(0.5, 7.0e-001, '--- Bitte Fermenter wählen ---', 'horizontalAlignment', 'center')
  ADM1DE Linearized : Subsystem  LoadFcn=adm1_loadfcn('ADM1DE');  mask(ADM1 implemented as DE system){fermenter_name=--- Bitte Fermenter wählen ---, initstate_type=--- Bitte Startzustandstyp wählen ---, datasource_type=--- Bitte Datenquelle wählen ---, savestate=off, isload=off, isbeingloaded=off, isbeingclosed=off, DEBUG_DISP=off}
      mask prompts: fermenter_name "name of the fermenter (fermenter_name)"; initstate_type "initial state type (initstate_type)"; datasource_type "source for the initial state (datasource_type)"; savestate "save final state in variable/file (overwrite existing type, except default, than save in user)"; isload "if checked then this block is loaded"; isbeingloaded "if checked then this block is actually being loaded"; isbeingclosed "if checked then this block is actually being closed"; DEBUG_DISP "if checked then DEBUG_DISP modus is on for this block"
      mask help:
      | This block is an implementation of the ADM1 as DE system as a clone of Simba's ADM1xp model.
      |
      | Remark: It is recommended to use the 'ADM1DE with GUI' block instead of this one, because the other block contains already measurement sensors, whose measurments are shown on a GUI.
      mask init: same as biogas/Anaerobic Digestion Models/Internal/ADM1DE
      settings: ModelCloseFcn=adm1_closefcn('ADM1DE');
      mask Help: eval('web( ''html/ADM1DE.html'', ''-helpbrowser'')')
      mask StyleString: popup(--- Bitte Fermenter wählen ---),popup(--- Bitte Startzustandstyp wählen ---|default|random|user),popup(--- Bitte Datenquelle wählen ---|file|workspace|extern|modelworkspace),checkbox,checkbox,checkbox,checkbox,checkbox
      mask CallbackString:
      | values= get_param(gcb, 'MaskValues');
      | 
      | if isempty(values)
      |     error('Could not read the parameter MaskValues of block %s!', gcb);
      | end
      | 
      | if strcmp( char(values(5,1)), 'on' )
      | 
      |     display_selected_fermenter(1, 0.7);
      | 
      | end
      | 
      | clear values;
      | |createinitstatetypepopup(2, 0);
      | |createdatasourcetypepopup(3, 0);
      | |||||
      mask Display:
      | image(imread('icon_s6_digester','bmp'),'center')
      | 
      | port_label('input',1,'Qin')
      | port_label('output',1,'Gas')
      | port_label('output',2,'Qe')
      | port_label('output',3,'int.vars')
      | text(0.5, 7.0e-001, '--- Bitte Fermenter wählen ---', 'horizontalAlignment', 'center')

== system biogas/Biogas Plant Components/Biogas Plant Name ==

== system biogas/Biogas Plant Components/Divider ==
  stream in : Inport
  Demux : Demux  Outputs=3
  divider : S-Function  FunctionName=divider  Parameters=n_outputs, splitVector  EnableBusSupport=off
      mask Help: eval('web( ''html/divider.html'', ''-helpbrowser'')')
  stream out1 : Outport
  stream out2 : Outport  Port=2
  stream out3 : Outport  Port=3
  wires:
  stream in/1 -> divider/1
  divider/1 -> Demux/1
  Demux/1 -> stream out1/1
  Demux/2 -> stream out2/1
  Demux/3 -> stream out3/1

== system biogas/Biogas Plant Components/Final Storage Tank ==
  ADM1 stream : Inport
  Terminator : Terminator
  final storage tank : S-Function  FunctionName=final_storage_tank  Parameters=sensors  EnableBusSupport=off
  wires:
  final storage tank/1 -> Terminator/1
  ADM1 stream/1 -> final storage tank/1

== system biogas/Biogas Plant Components/Get Data of Sensors Object ==
  Constant : Constant
  sensor_data : S-Function  FunctionName=sensor_data  Parameters=sensors, processvalue, id_in_array, index, noisy, substrate  EnableBusSupport=off
  value : Outport
  wires:
  Constant/1 -> sensor_data/1
  sensor_data/1 -> value/1

== system biogas/Biogas Plant Components/Hydraulic Delay ==
  ADM1 stream : Inport
  hydraulic delay : S-Function  FunctionName=hydraulic_delay  Parameters=DEBUG, plant, char(plant.getDigesterID(fermenter_name_start - 1)), char(plant.getDigesterID(fermenter_name_destiny - 1)), initstatetypes(initstate_type - 1), datasourcetypes(datasource_type - 1), savestate, time_constant, V_min  EnableBusSupport=off
  stream : Outport
  wires:
  ADM1 stream/1 -> hydraulic delay/1
  hydraulic delay/1 -> stream/1

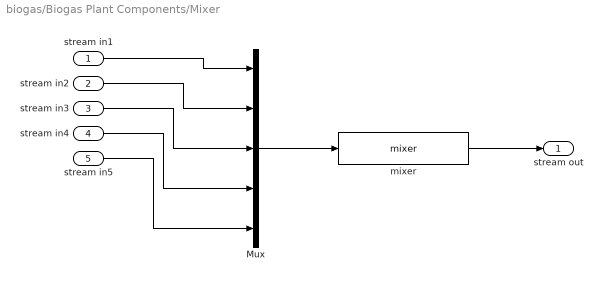
== system biogas/Biogas Plant Components/Mixer ==
  stream in1 : Inport
  stream in2 : Inport  Port=2
  stream in3 : Inport  Port=3
  stream in4 : Inport  Port=4
  stream in5 : Inport  Port=5
  Mux : Mux  Inputs=5
  mixer : S-Function  FunctionName=mixer  Parameters=n_inputs  EnableBusSupport=off
      mask Help: eval('web( ''html/mixer.html'', ''-helpbrowser'')')
  stream out : Outport
  wires:
  mixer/1 -> stream out/1
  Mux/1 -> mixer/1
  stream in1/1 -> Mux/1
  stream in2/1 -> Mux/2
  stream in3/1 -> Mux/3
  stream in4/1 -> Mux/4
  stream in5/1 -> Mux/5
